simulink subsystem "Reference"  (R2023a)
settings: Solver=VariableStepAuto  StartTime=0.0  StopTime=10.0  RelTol=1e-3
settings Model: Creator=jipva  LastModifiedBy=jipva

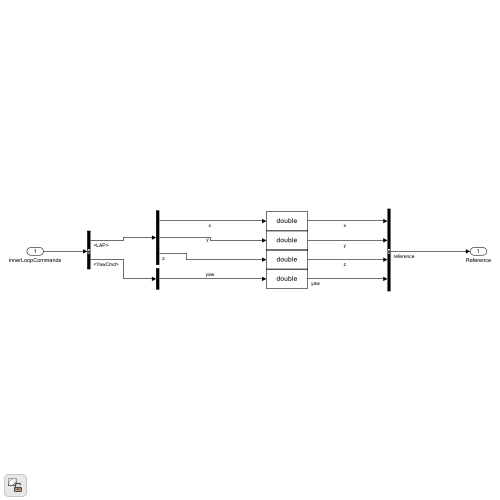
[thumbnail: Simulink's stored preview of the top-level diagram]
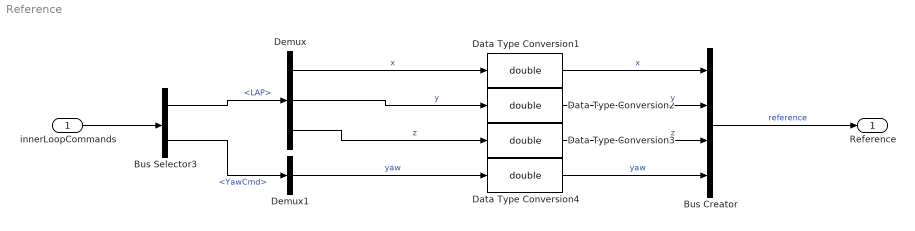
== system Reference ==
  innerLoopCommands : Inport
  Bus Creator : BusCreator  Inputs=4
  Bus Selector3 : BusSelector  OutputSignals=LAP,YawCmd
  Data Type Conversion{1..4} (4 alike) : DataTypeConversion  OutDataTypeStr=double  SaturateOnIntegerOverflow=off  RndMeth=Floor
  Demux : Demux  Outputs=3
  Demux1 : Demux  Outputs=1
  Reference : Outport
  wires:
  Data Type Conversion2/1 -> Bus Creator/2  "y"
  Demux1/1 -> Data Type Conversion4/1  "yaw"
  Data Type Conversion3/1 -> Bus Creator/3  "z"
  Data Type Conversion1/1 -> Bus Creator/1  "x"
  Data Type Conversion4/1 -> Bus Creator/4  "yaw"
  Demux/1 -> Data Type Conversion1/1  "x"
  Demux/2 -> Data Type Conversion2/1  "y"
  Demux/3 -> Data Type Conversion3/1  "z"
  innerLoopCommands/1 -> Bus Selector3/1
  Bus Creator/1 -> Reference/1  "reference"
  Bus Selector3/1 -> Demux/1  "<LAP>"
  Bus Selector3/2 -> Demux1/1  "<YawCmd>"
